simulink model "Part1B"  (R2024a)
settings: Solver=VariableStepAuto  StartTime=0.0  StopTime=10.0  RelTol=1e-3
settings Model: Creator=kyleo  LastModifiedBy=kyleo

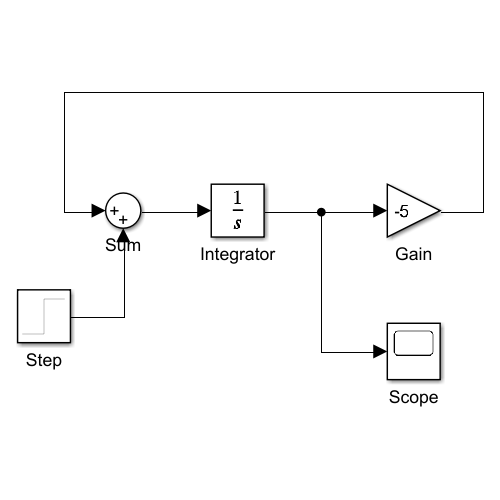
[thumbnail: Simulink's stored preview of the top-level diagram]
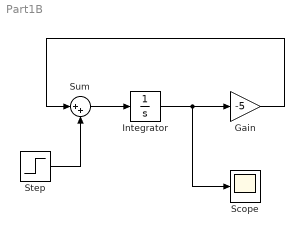
== system Part1B ==
  Gain : Gain  Gain=-5
  Integrator : Integrator  InitialCondition=-2
  Scope : Scope
  Step : Step  SampleTime=0
  Sum : Sum  Inputs=|++
  wires:
  Integrator/1 -> Scope/1, Gain/1
  Gain/1 -> Sum/1
  Step/1 -> Sum/2
  Sum/1 -> Integrator/1
